simulink model "simulateQPSK"  (R2017a)
settings: Solver=VariableStepAuto  StartTime=0.0  StopTime=100  RelTol=1e-3
InitFcn:
  | T_bit = 1/1000;        % bit time
  | T_sym = T_bit * 2;   % QPSK encodes 2 bits per symbol
libraries: commutil2 x2, commsink2 x2, commdigbbndpm3 x2, commchan3 x1, commrandsrc3 x1
settings Model: Creator=prust  LastModifiedBy=prust

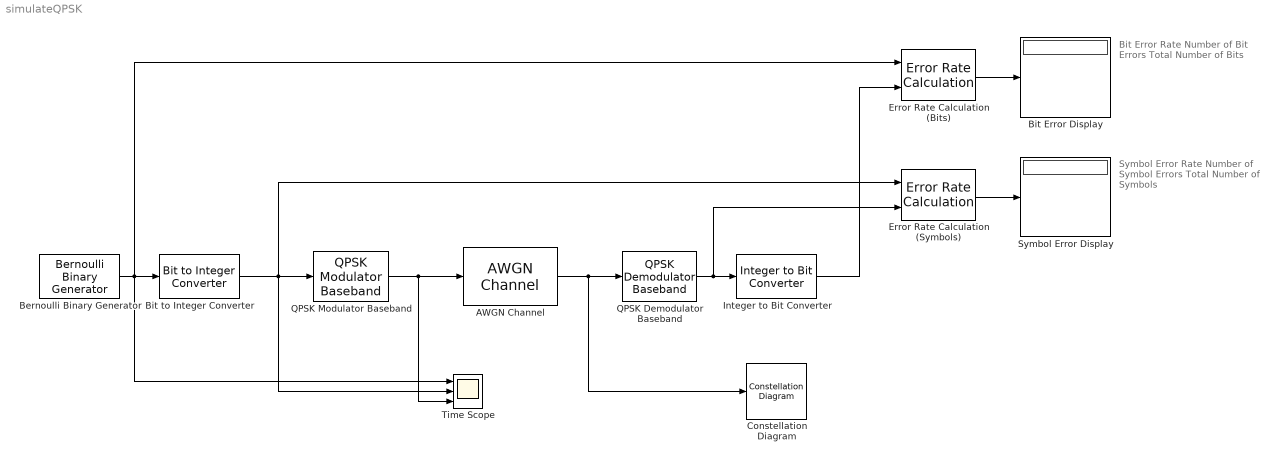
== system simulateQPSK ==
  note: Symbol Error Rate
      |
      | Number of Symbol Errors
      |
      | Total Number of Symbols
  note: Bit Error Rate
      |
      | Number of Bit Errors
      |
      | Total Number of Bits
  AWGN Channel : commchan3/AWGN Channel  InputProcessing=Columns as channels (frame based)  seed=67  noiseMode="Signal to noise ratio  (Eb/No)"  EbNodB=4  EsNodB=10  SNRdB=10  bitsPerSym=2  Ps=1  Tsym=T_sym  variance=1
  Bernoulli Binary Generator : commrandsrc3/Bernoulli Binary Generator  ProbabilityOfZero=0.5  SeedSource=Auto  Seed=0  SampleTime=T_bit  SamplesPerFrame=1000  OutputDataType=double  SimulateUsing=Interpreted execution
  Bit Error Display : Display
  Bit to Integer Converter : commutil2/Bit to Integer Converter  nbits=2  bitOrder=MSB first  signedOutputValues=Unsigned  outDtype=Inherit via internal rule  outDtypeSigned=Inherit via internal rule
  Constellation Diagram : ConstellationDiagram
  Error Rate Calculation (Bits) : commsink2/Error Rate Calculation  N=0  st_delay=0  cp_mode=Entire frame  subframe=[]  PMode=Port  WsName=ErrorVec  RsMode2=off  stop=off  numErr=100  maxBits=1e6
  Error Rate Calculation (Symbols) : commsink2/Error Rate Calculation  N=0  st_delay=0  cp_mode=Entire frame  subframe=[]  PMode=Port  WsName=ErrorVec  RsMode2=off  stop=off  numErr=100  maxBits=1e6
  Integer to Bit Converter : commutil2/Integer to Bit Converter  nbits=2  signedInputValues=Unsigned  bitOrder=MSB first  outDtype=Inherit via internal rule
  QPSK Demodulator Baseband : commdigbbndpm3/QPSK Demodulator Baseband  OutType=Integer  DecType=Hard decision  VarSource=Dialog  Variance=1  Dec=Gray  Ph=pi/4  outDtype1=Inherit via internal rule  outDtype2=Inherit via internal rule  derotateFactorWordLen=16  derotateFactorDataTypeStr=Inherit: Same word length as input  derotateFactorLastDataTypeStr=Inherit: Same word length as input
  QPSK Modulator Baseband : commdigbbndpm3/QPSK Modulator Baseband  InType=Integer  Enc=Gray  Ph=pi/4  outDtype=double  outWordLen=16  outUDDataType=sfix(16)  outFracLenMode=Best precision  outFracLen=15  outDataTypeStr=double  outLastDataTypeStr=double
  Symbol Error Display : Display
  Time Scope : Scope  NumInputPorts=3
  wires:
  Bit to Integer Converter/1 -> Time Scope/2, QPSK Modulator Baseband/1, Error Rate Calculation (Symbols)/1
  QPSK Modulator Baseband/1 -> Time Scope/3, AWGN Channel/1
  AWGN Channel/1 -> QPSK Demodulator Baseband/1, Constellation Diagram/1
  QPSK Demodulator Baseband/1 -> Error Rate Calculation (Symbols)/2, Integer to Bit Converter/1
  Error Rate Calculation (Symbols)/1 -> Symbol Error Display/1
  Bernoulli Binary Generator/1 -> Error Rate Calculation (Bits)/1, Time Scope/1, Bit to Integer Converter/1
  Integer to Bit Converter/1 -> Error Rate Calculation (Bits)/2
  Error Rate Calculation (Bits)/1 -> Bit Error Display/1
